simulink model "pendulum_without_filter"  (R2020b)
settings: Solver=FixedStepAuto  StartTime=0.0  StopTime=10  FixedStep=1e-3  RelTol=1e-3
values from neighbouring files (symbols this model uses):
  controlador = projetarControlador(requisitos, planta)    [executarTudo.m]    (also in runAll.m; simular.m)
  planta = obterPlanta()    [codetest.m]    (also in executarTudo.m; nextState.m; runAll.m; simular.m)
  thetar = 0    [executarTudo.m]    (also in runAll.m)
undefined symbols (not defined in the file or in its folder): varCom, varMed
libraries: pid_lib x1
settings Model: Creator=davi  LastModifiedBy=alexandremaranhao

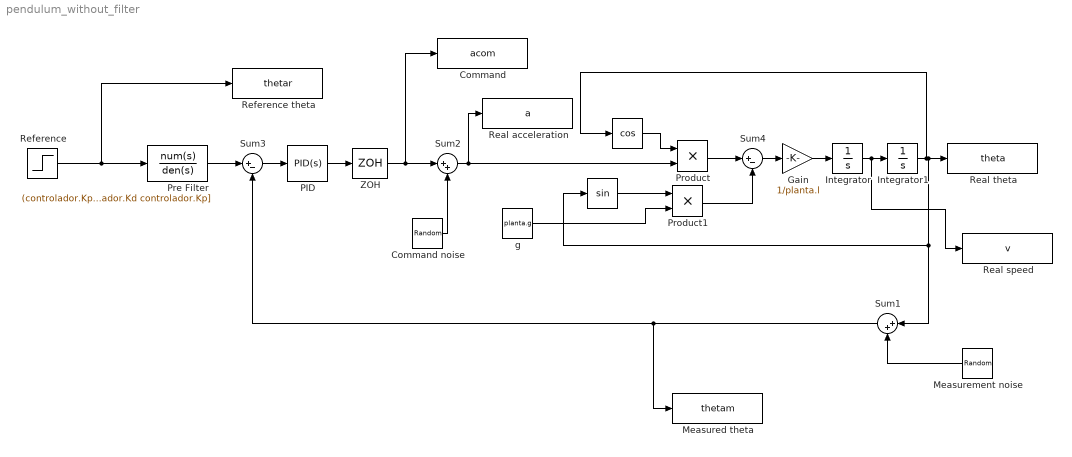
== system pendulum_without_filter ==
  " " : Trigonometry  Operator=cos
  "  " : Trigonometry
  Command : ToWorkspace  VariableName=acom  SaveFormat=Structure With Time  SampleTime=-1
  Command noise : RandomNumber  Variance=varCom  SampleTime=1e-2
  Gain : Gain  Gain=1/planta.l
  Integrator : Integrator
  Integrator1 : Integrator
  Measured theta : ToWorkspace  VariableName=thetam  SaveFormat=Structure With Time  SampleTime=-1
  Measurement noise : RandomNumber  Variance=varMed  SampleTime=1e-2
  PID : pid_lib/PID Controller  Controller=PID  Form=Parallel  TimeDomain=Continuous-time  UseExternalTs=off  SampleTime=1e-2  IntegratorMethod=Forward Euler  FilterMethod=Forward Euler  ControllerParametersSource=internal  P=controlador.Kp  I=0  D=controlador.Kd  UseFilter=on  N=100  TunerSelectOption=Transfer Function Based (PID Tuner App)  InitialConditionSource=internal  InitialConditionForIntegrator=0  InitialConditionForFilter=0  DifferentiatorICPrevScaledInput=0  ExternalReset=none  TrackingMode=off  Kt=1  LimitOutput=off  SatLimitsSource=internal  UpperSaturationLimit=inf  LowerSaturationLimit=-inf  LinearizeAsGain=on  AntiWindupMode=none  Kb=1  POutMin=[]  POutMax=[]  IOutMin=[]  IOutMax=[]  DOutMin=[]  DOutMax=[]  NOutMin=[]  NOutMax=[]  SumOutMin=[]  SumOutMax=[]  SaturationOutMin=[]  SaturationOutMax=[]  PParamMin=[]  PParamMax=[]  IParamMin=[]  IParamMax=[]  DParamMin=[]  DParamMax=[]  NParamMin=[]  NParamMax=[]  KbParamMin=[]  KbParamMax=[]  KtParamMin=[]  KtParamMax=[]  KbOutMin=[]  KbOutMax=[]  KtOutMin=[]  KtOutMax=[]  IntegratorOutMin=[]  IntegratorOutMax=[]  FilterOutMin=[]  FilterOutMax=[]  SumI1OutMin=[]  SumI1OutMax=[]  SumI2OutMin=[]  SumI2OutMax=[]  SumI3OutMin=[]  SumI3OutMax=[]  SumI4OutMin=[]  SumI4OutMax=[]  SumDOutMin=[]  SumDOutMax=[]  DifferentiatorOutMin=[]  DifferentiatorOutMax=[]  FilterDiffOutCoefMin=[]  FilterDiffOutCoefMax=[]  ReciprocalOutMin=[]  ReciprocalOutMax=[]  SumDenOutMin=[]  SumDenOutMax=[]  SumNumOutMin=[]  SumNumOutMax=[]  DivideOutMin=[]  DivideOutMax=[]  UdiffTsProdOutMin=[]  UdiffTsProdOutMax=[]  NTsProdOutMin=[]  NTsProdOutMax=[]  UintegralTsProdOutMin=[]  UintegralTsProdOutMax=[]  UngainTsProdOutMin=[]  UngainTsProdOutMax=[]  IntegratorContinuousStateAttributes=''  IntegratorStateMustResolveToSignalObject=off  IntegratorRTWStateStorageClass=Auto  FilterContinuousStateAttributes=''  FilterStateMustResolveToSignalObject=off  FilterRTWStateStorageClass=Auto  ParallelPVariant=InternalParameters  IdealPVariant=Disabled  IVariant=InternalParameters  DVariant=InternalParameters  IntegratorVariant=Continuous  SatVariant=Disabled  AWVariant=Passthrough  PCopyVariant=Disabled  TRVariant=Disabled  FdbkBlocksVariant=Forward  IdealPFdbkVariant=Disabled  SatFdbkVariant=Disabled  DerivativeFilterVariant=ContFilter  NVariant=InternalParameters  NCopyVariant=Disabled  FilterICVariant=InternalICsFilter  IntegratorICVariant=InternalICs  ExternalResetVariant=Disabled  TRSumVariant=Passthrough  SumFdbkVariant=Disabled  SumVariant=Sum_PID  TsampFilterVariant=InternalTs  TsampNgainVariant=Passthrough  TsampIntegralVariant=Passthrough  ExternalSaturationOutDataTypeStr=Inherit: Same as second input
  Pre Filter : TransferFcn  Numerator=(controlador.Kp+planta.g)  Denominator=[controlador.Kd controlador.Kp]
  Product : Product
  Product1 : Product
  Real acceleration : ToWorkspace  VariableName=a  SaveFormat=Structure With Time  SampleTime=-1
  Real speed : ToWorkspace  VariableName=v  SaveFormat=Structure With Time  SampleTime=-1
  Real theta : ToWorkspace  VariableName=theta  SaveFormat=Structure With Time  SampleTime=-1
  Reference : Step  Time=0  After=thetar  SampleTime=0
  Reference theta : ToWorkspace  VariableName=thetar  SaveFormat=Structure With Time  SampleTime=-1
  Sum1 : Sum  Inputs=|++
  Sum2 : Sum  Inputs=|++
  Sum3 : Sum  Inputs=|+-
  Sum4 : Sum  Inputs=|+-
  ZOH : ZeroOrderHold  SampleTime=1e-2
  g : Constant  Value=planta.g
  wires:
  Product/1 -> Sum4/1
  Measurement noise/1 -> Sum1/2
  Sum2/1 -> Product/2, Real acceleration/1
  Command noise/1 -> Sum2/2
  Reference/1 -> Pre Filter/1, Reference theta/1
  Pre Filter/1 -> Sum3/1
  " "/1 -> Product/1
  "  "/1 -> Product1/1
  g/1 -> Product1/2
  Product1/1 -> Sum4/2
  Sum4/1 -> Gain/1
  Gain/1 -> Integrator/1
  Integrator/1 -> Real speed/1, Integrator1/1
  Integrator1/1 -> "  "/1, Sum1/1, Real theta/1, " "/1
  Sum3/1 -> PID/1
  Sum1/1 -> Sum3/2, Measured theta/1
  PID/1 -> ZOH/1
  ZOH/1 -> Command/1, Sum2/1
